simulink model "simulation_9209"  (R2019a)
settings: Solver=VariableStepAuto  StartTime=0.0  StopTime=20  RelTol=1e-3
libraries: simulink x3, fuzblock x1
settings Model: Creator=kosta  LastModifiedBy=kosta
settings DebuggingCC: ParameterPrecisionLossMsg=none

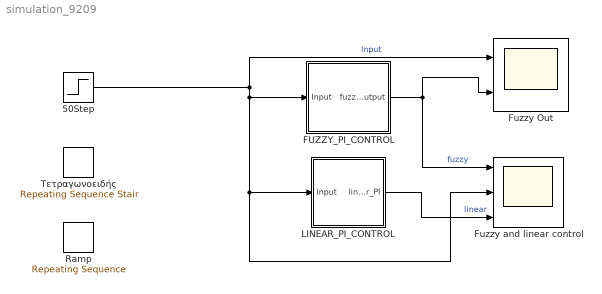
== system simulation_9209 ==
  "50Step " : Step  After=50  SampleTime=0
  FUZZY_PI_CONTROL : Subsystem
  "Fuzzy Out " : Scope  NumInputPorts=2
  Fuzzy and linear control : Scope  NumInputPorts=3
  LINEAR_PI_CONTROL : Subsystem
  Ramp : simulink/Sources/Repeating Sequence  rep_seq_t=[0 5 10 20]  rep_seq_y=[0 50 50 0]
  Τετραγωνοειδής : simulink/Sources/Repeating Sequence Stair  OutValues=[50 50 50 50 50 20 20 20 20 20 40 40 40 40 40 40 40 40 40 40 ].'  tsamp=1  OutMin=[]  OutMax=[]  OutDataTypeStr=double  OutputDataTypeScalingMode=double  OutDataType=fixdt(0,8)  ConRadixGroup=Best Precision: Vector-wise  OutScaling=2^-12
  wires:
  FUZZY_PI_CONTROL/1(fuzzy output) -> Fuzzy and linear control/1, "Fuzzy Out "/2  "fuzzy"
  LINEAR_PI_CONTROL/1(linear_PI) -> Fuzzy and linear control/3  "linear"
  "50Step "/1 -> "Fuzzy Out "/1, Fuzzy and linear control/2, LINEAR_PI_CONTROL/1(Input), FUZZY_PI_CONTROL/1(Input)  "Input"

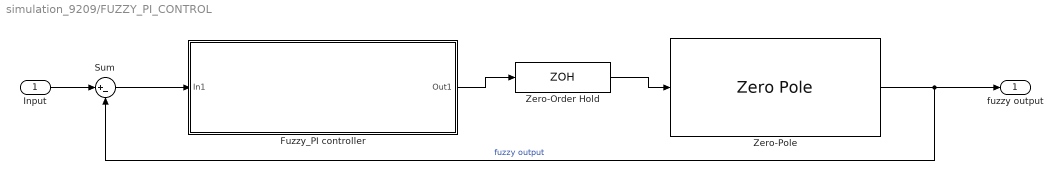
== system simulation_9209/FUZZY_PI_CONTROL ==
  Input : Inport
  Fuzzy_PI controller : Subsystem
  Sum : Sum  Inputs=|+-
  Zero-Order Hold : ZeroOrderHold  SampleTime=0.01
  Zero-Pole : ZeroPole  Zeros=[]  Poles=[-0.1 -10]  Gain=25
  fuzzy output : Outport
  wires:
  Zero-Order Hold/1 -> Zero-Pole/1
  Zero-Pole/1 -> fuzzy output/1, Sum/2  "fuzzy output"
  Fuzzy_PI controller/1(Out1) -> Zero-Order Hold/1
  Input/1 -> Sum/1
  Sum/1 -> Fuzzy_PI controller/1(In1)

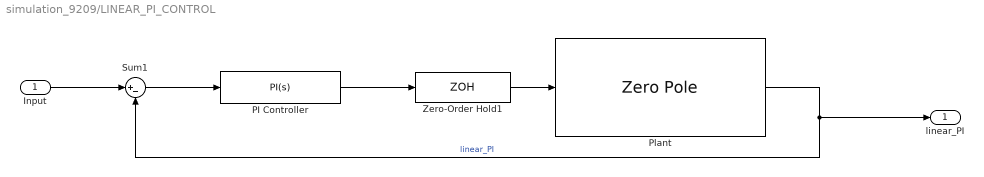
== system simulation_9209/LINEAR_PI_CONTROL ==
  Input : Inport
  PI Controller : simulink/Continuous/PID Controller  Controller=PI  Form=Parallel  TimeDomain=Continuous-time  SampleTime=0.01  IntegratorMethod=Forward Euler  FilterMethod=Forward Euler  ControllerParametersSource=internal  P=1.85  I=0.5  D=0  UseFilter=on  N=100  TunerSelectOption=Transfer Function Based (PID Tuner App)  InitialConditionSource=internal  InitialConditionForIntegrator=0  InitialConditionForFilter=0  DifferentiatorICPrevScaledInput=0  ExternalReset=none  TrackingMode=off  Kt=1  LimitOutput=off  UpperSaturationLimit=inf  LowerSaturationLimit=-inf  LinearizeAsGain=on  AntiWindupMode=none  Kb=1  POutMin=[]  POutMax=[]  IOutMin=[]  IOutMax=[]  DOutMin=[]  DOutMax=[]  NOutMin=[]  NOutMax=[]  SumOutMin=[]  SumOutMax=[]  SaturationOutMin=[]  SaturationOutMax=[]  PParamMin=[]  PParamMax=[]  IParamMin=[]  IParamMax=[]  DParamMin=[]  DParamMax=[]  NParamMin=[]  NParamMax=[]  KbParamMin=[]  KbParamMax=[]  KtParamMin=[]  KtParamMax=[]  KbOutMin=[]  KbOutMax=[]  KtOutMin=[]  KtOutMax=[]  IntegratorOutMin=[]  IntegratorOutMax=[]  FilterOutMin=[]  FilterOutMax=[]  SumI1OutMin=[]  SumI1OutMax=[]  SumI2OutMin=[]  SumI2OutMax=[]  SumI3OutMin=[]  SumI3OutMax=[]  SumI4OutMin=[]  SumI4OutMax=[]  SumDOutMin=[]  SumDOutMax=[]  DifferentiatorOutMin=[]  DifferentiatorOutMax=[]  FilterDiffOutCoefMin=[]  FilterDiffOutCoefMax=[]  ReciprocalOutMin=[]  ReciprocalOutMax=[]  SumDenOutMin=[]  SumDenOutMax=[]  SumNumOutMin=[]  SumNumOutMax=[]  DivideOutMin=[]  DivideOutMax=[]  IntegratorContinuousStateAttributes=''  IntegratorStateMustResolveToSignalObject=off  IntegratorRTWStateStorageClass=Auto  FilterContinuousStateAttributes=''  FilterStateMustResolveToSignalObject=off  FilterRTWStateStorageClass=Auto  ParallelPVariant=InternalParameters  IdealPVariant=Disabled  IVariant=InternalParameters  DVariant=Disabled  IntegratorVariant=Continuous  SatVariant=Disabled  AWVariant=Passthrough  PCopyVariant=Disabled  TRVariant=Disabled  FdbkBlocksVariant=Forward  IdealPFdbkVariant=Disabled  SatFdbkVariant=Disabled  DerivativeFilterVariant=Disabled  NVariant=Disabled  NCopyVariant=Disabled_SignalSpec  FilterICVariant=Disabled  IntegratorICVariant=InternalICs  ExternalResetVariant=Disabled  TRSumVariant=Passthrough  SumFdbkVariant=Disabled  SumVariant=Sum_PI
  Plant : ZeroPole  Zeros=[]  Poles=[-0.1 -10]  Gain=25
  Sum1 : Sum  Inputs=|+-
  Zero-Order Hold1 : ZeroOrderHold  SampleTime=0.01
  linear_PI : Outport
  wires:
  PI Controller/1 -> Zero-Order Hold1/1
  Zero-Order Hold1/1 -> Plant/1
  Sum1/1 -> PI Controller/1
  Plant/1 -> Sum1/2, linear_PI/1  "linear_PI"
  Input/1 -> Sum1/1

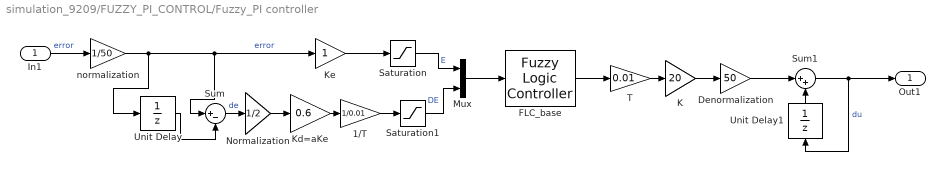
== system simulation_9209/FUZZY_PI_CONTROL/Fuzzy_PI controller ==
  In1 : Inport
  1/T : Gain  Gain=1/0.01
  Denormalization : Gain  Gain=50
  FLC_base : fuzblock/Fuzzy Logic  Controller  FIS=FLC_base  OutputSampleNumber=101  DataType=single  FuzzifiedInputs=off  RuleFiringStrengths=off  RuleOutputs=off  AggregatedOutputs=off  SimulateUsing=Interpreted execution  OutOfRangeInputValueMessage=none  NoRuleFiredMessage=none  EmptyOutputFuzzySetMessage=warning
  K : Gain  Gain=20
  Kd=aKe : Gain  Gain=0.6
  Ke : Gain
  Mux : Mux  Inputs=2
  Normalization : Gain  Gain=1/2
  Saturation : Saturate  UpperLimit=1  LowerLimit=-1
  Saturation1 : Saturate  UpperLimit=1  LowerLimit=-1
  Sum : Sum  Inputs=|+-
  Sum1 : Sum  Inputs=|++
  T : Gain  Gain=0.01
  Unit Delay : UnitDelay  SampleTime=-1  HasFrameUpgradeWarning=on
  Unit Delay1 : UnitDelay  SampleTime=-1  HasFrameUpgradeWarning=on
  normalization : Gain  Gain=1/50
  Out1 : Outport
  wires:
  Unit Delay/1 -> Sum/2
  Ke/1 -> Saturation/1
  K/1 -> Denormalization/1
  Mux/1 -> FLC_base/1
  Saturation/1 -> Mux/1  "E"
  Saturation1/1 -> Mux/2  "DE"
  FLC_base/1 -> T/1
  T/1 -> K/1
  Sum1/1 -> Out1/1, Unit Delay1/1  "du"
  Denormalization/1 -> Sum1/1
  Unit Delay1/1 -> Sum1/2
  In1/1 -> normalization/1  "error"
  1/T/1 -> Saturation1/1
  Kd=aKe/1 -> 1/T/1
  Sum/1 -> Normalization/1  "de"
  normalization/1 -> Sum/1, Ke/1, Unit Delay/1  "error"
  Normalization/1 -> Kd=aKe/1
